simulink model "sampleModel169"  (R2021b)
settings: Solver=VariableStepAuto  StartTime=0.0  StopTime=10.0  RelTol=1e-3
libraries: simulink x3
settings Model: Creator=user  LastModifiedBy=user

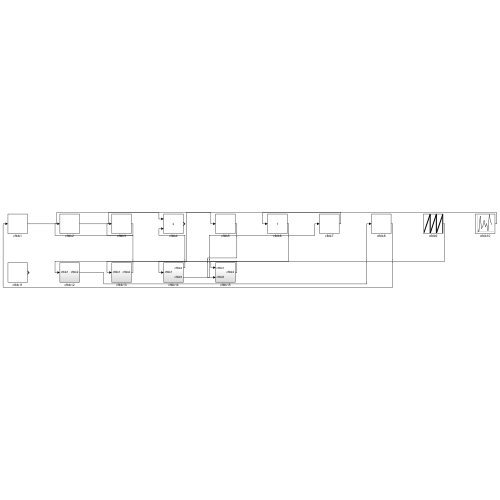
[thumbnail: Simulink's stored preview of the top-level diagram]
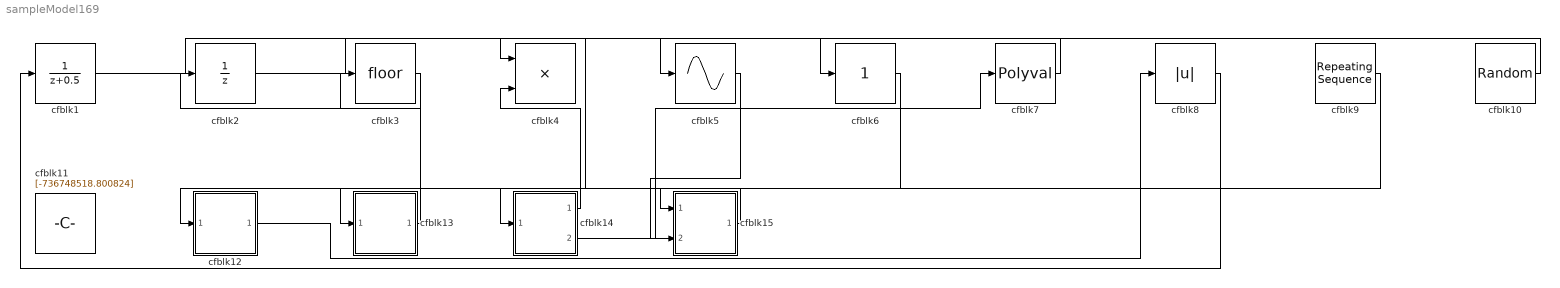
== system sampleModel169 ==
  cfblk1 : DiscreteTransferFcn  SampleTime=1
  cfblk10 : UniformRandomNumber  Minimum=[-814846663.886244]  Maximum=[2969662637.402277]  Seed=[51641665.000000]  SampleTime=0.1
  cfblk11 : Constant  Value=[-736748518.800824]  SampleTime=1
  cfblk12 : Subsystem
  cfblk13 : Subsystem
  cfblk14 : Subsystem
  cfblk15 : Subsystem
  cfblk2 : UnitDelay  HasFrameUpgradeWarning=on
  cfblk3 : Rounding
  cfblk4 : Product
  cfblk5 : Sin  TimeSource=Use external signal  SampleTime=0
  cfblk6 : simulink/Math Operations/Slider Gain  gain=1  low=0  high=2
  cfblk7 : Polyval  Coefs=[ +2.081618890e-019, -1.441693666e-014, +4.719686976e-010, -8.536869453e-006, +1.621573104e-001, -8.087801117e+001 ]
  cfblk8 : Abs
  cfblk9 : simulink/Sources/Repeating Sequence  rep_seq_t=[0 2]  rep_seq_y=[-609049862.992422, 855860176.653759]
  wires:
  cfblk6/1 -> cfblk15/1(cfblk1)
  cfblk5/1 -> cfblk15/2(cfblk5)
  cfblk1/1 -> cfblk4/1
  cfblk10/1 -> cfblk13/1(cfblk1)
  cfblk7/1 -> cfblk6/1
  cfblk12/1(cfblk2) -> cfblk8/1
  cfblk2/1 -> cfblk5/1
  cfblk3/1 -> cfblk2/1
  cfblk8/1 -> cfblk1/1
  cfblk9/1 -> cfblk14/1(cfblk1)
  cfblk14/1(cfblk2) -> cfblk4/2
  cfblk13/1(cfblk2) -> cfblk3/1
  cfblk14/2(cfblk5) -> cfblk7/1
  cfblk15/1(cfblk2) -> cfblk12/1(cfblk1)

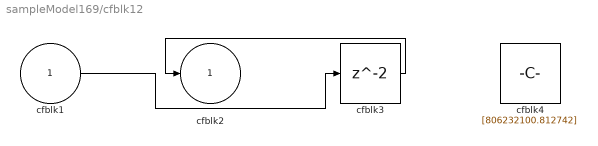
== system sampleModel169/cfblk12 ==
  cfblk1 : Inport
  cfblk3 : Delay  SampleTime=1
  cfblk4 : Constant  Value=[806232100.812742]  SampleTime=1
  cfblk2 : Outport
  wires:
  cfblk3/1 -> cfblk2/1
  cfblk1/1 -> cfblk3/1

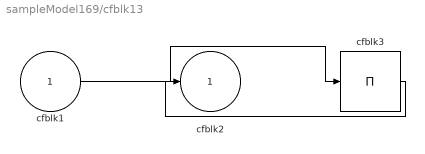
== system sampleModel169/cfblk13 ==
  cfblk1 : Inport
  cfblk3 : Product  Inputs=*
  cfblk2 : Outport
  wires:
  cfblk1/1 -> cfblk3/1
  cfblk3/1 -> cfblk2/1

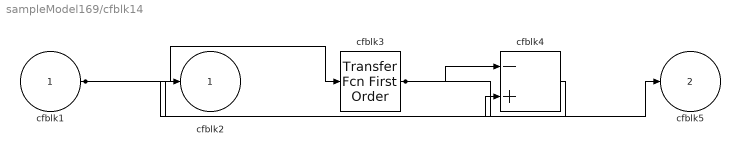
== system sampleModel169/cfblk14 ==
  cfblk1 : Inport
  cfblk3 : simulink/Discrete/Transfer Fcn First Order  PoleZ=0.95  ICPrevOutput=0.0  DoSatur=off
  cfblk4 : Sum  Inputs=-+
  cfblk2 : Outport
  cfblk5 : Outport  Port=2
  wires:
  cfblk1/1 -> cfblk3/1, cfblk4/2
  cfblk3/1 -> cfblk4/1, cfblk5/1
  cfblk4/1 -> cfblk2/1

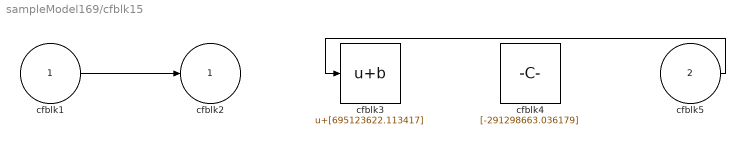
== system sampleModel169/cfblk15 ==
  cfblk1 : Inport
  cfblk5 : Inport  Port=2
  cfblk3 : Bias  Bias=[695123622.113417]
  cfblk4 : Constant  Value=[-291298663.036179]  SampleTime=1
  cfblk2 : Outport
  wires:
  cfblk1/1 -> cfblk2/1
  cfblk5/1 -> cfblk3/1
